simulink subsystem "PWMOsc"  (R2024a)
settings: Solver=VariableStepAuto  StartTime=0.0  StopTime=10.0  RelTol=1e-3
undefined symbols (not defined in the file or in its folder): vmax, vmin
settings Model: Creator=dfurodet  LastModifiedBy=david
settings RTWCC: GPUComputeCapability=3.5

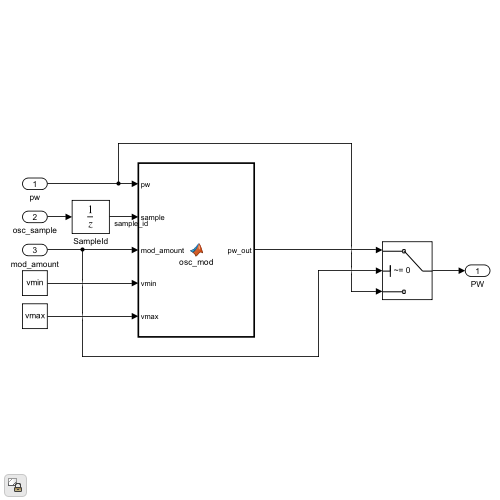
[thumbnail: Simulink's stored preview of the top-level diagram]
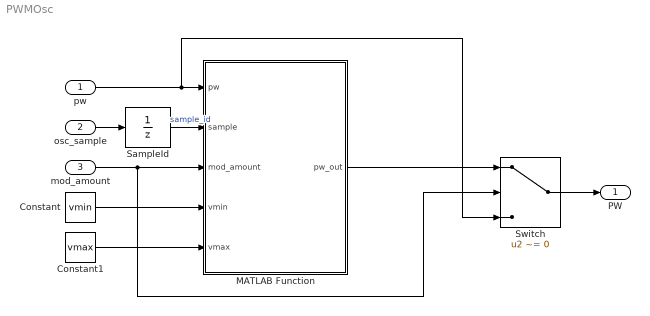
== system PWMOsc ==
  pw : Inport
  osc_sample : Inport  Port=2
  mod_amount : Inport  Port=3
  Constant : Constant  Value=vmin
  Constant1 : Constant  Value=vmax
  MATLAB Function : MATLAB Function  TreatAsAtomicUnit=on
  SampleId : UnitDelay  HasFrameUpgradeWarning=on
  Switch : Switch  Criteria=u2 ~= 0  SaturateOnIntegerOverflow=off  InputSameDT=off
  PW : Outport
  wires:
  pw/1 -> MATLAB Function/1(pw), Switch/3
  osc_sample/1 -> SampleId/1
  Switch/1 -> PW/1
  MATLAB Function/1(pw_out) -> Switch/1
  mod_amount/1 -> MATLAB Function/3(mod_amount), Switch/2
  SampleId/1 -> MATLAB Function/2(sample)  "sample_id"
  Constant/1 -> MATLAB Function/4(vmin)
  Constant1/1 -> MATLAB Function/5(vmax)

== matlab function PWMOsc/MATLAB Function ==
  data: pw input; pw_out output; sample input; mod_amount input; vmin input; vmax input
function pw_out = osc_mod(pw, sample, mod_amount, vmin, vmax)
amplitude = vmax - vmin;
amount = double(mod_amount) * sample / 100;
normd = (amount - vmin);
pw_out = pw * normd / amplitude;
